simulink model "s6_template"  (R2023b)
settings: Solver=ode4  StartTime=0.0  StopTime=inf  FixedStep=P_sim_dt  RelTol=1e-3
InitFcn:
  | s6_data;
values from neighbouring files (symbols this model uses):
  CarInputsCmdForward = uint8(1)    [p_mad_car.m]
  CarInputsCmdHalt = uint8(0)    [p_mad_car.m]
  CarInputsCmdReverse = uint8(2)    [p_mad_car.m]
  CarInputsCmdSlow = uint8(3)    [p_mad_car.m]
  P_p_Bf = 0.7    [p_mad_car.m]
  P_p_Br = 0.7    [p_mad_car.m]
  P_p_Cf = 2    [p_mad_car.m]
  P_p_Cr = 2    [p_mad_car.m]
  P_p_delta_max = 21.58/180*pi    (= 0.37664205258)    [p_mad_car.m]
  P_p_Df = 2    [p_mad_car.m]
  P_p_Dr = 2.5    [p_mad_car.m]
  P_p_Ef = -0.1    [p_mad_car.m]
  P_p_Er = -0.05    [p_mad_car.m]
  P_p_J = 192e-6    (= 0.000192)    [p_mad_car.m]
  P_p_k = 2.51    [p_mad_car.m]
  P_p_l = abs(P_p_frontaxle_1 + P_p_rearaxle_1)    [p_mad_car.m]
  P_p_lf = P_p_frontaxle_1    (= 0.05)    [p_mad_car.m]
  P_p_lr = P_p_rearaxle_1    (= 0.049)    [p_mad_car.m]
  P_p_m = 132e-3    (= 0.132)    [p_mad_car.m]
  P_p_T = 316e-3    (= 0.316)    [p_mad_car.m]
  P_p_Tt = P_p_uTt + P_p_output_Tt    (= 0.1)    [p_mad_car.m]
libraries: mad_lib_template x1
settings Model: Creator=hmekiedj  LastModifiedBy=Dominik
settings SolverCC: AlgebraicLoopSolver=TrustRegion
settings DataIOCC: ReturnWorkspaceOutputs=off
settings DebuggingCC: UnconnectedInputMsg=warning  UnconnectedOutputMsg=warning  UnconnectedLineMsg=warning  ArithmeticOperatorsInVariantConditions=warning
settings ModelReferenceCC: EnableRefExpFcnMdlSchedulingChecks=on
settings SFSimCC: SimUseLocalCustomCode=off  CustomCodeUndefinedFunction=UseInterfaceOnly
settings RTWCC: RTWUseLocalCustomCode=off  DLArmComputeVersion=19.05
settings CodeAppCC: StateflowObjectComments=on

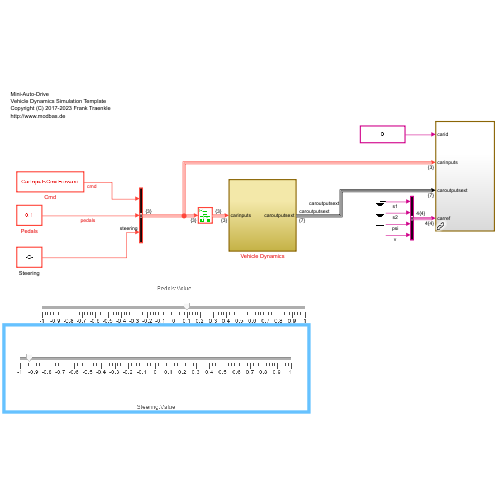
[thumbnail: Simulink's stored preview of the top-level diagram]
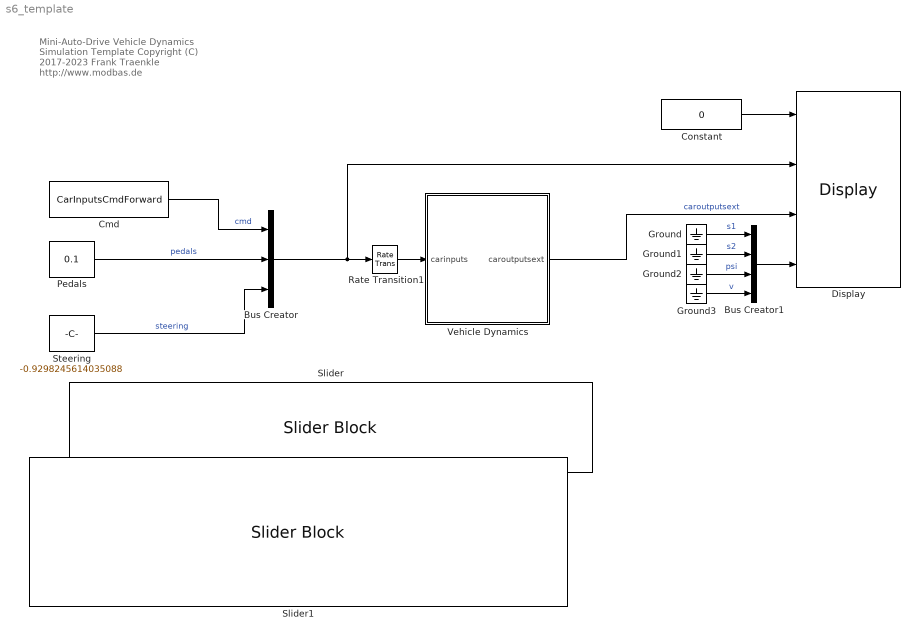
== system s6_template ==
  note: Mini-Auto-Drive
      | Vehicle Dynamics Simulation Template
      | Copyright (C) 2017-2023 Frank Traenkle
      | http://www.modbas.de
  Bus Creator : BusCreator  Inputs=3
  Bus Creator1 : BusCreator  Inputs=4
  Cmd : Constant  Value=CarInputsCmdForward  SampleTime=-1
  Constant : Constant  Value=0
  Display : mad_lib_template/Display  SystemSampleTime=-1  VariantActivationTime=update diagram  AllowFlexibleInterface=on  Latency=0  AutoFrameSizeCalculation=off
  Ground{,1..3} (4 alike) : Ground
  Pedals : Constant  Value=0.1  SampleTime=-1
  Rate Transition1 : RateTransition
  Slider : SliderBlock  ScaleMin=-1  ScaleMax=1
  Slider1 : SliderBlock  LabelPosition=Bottom  ScaleMin=-1  ScaleMax=1
  Steering : Constant  Value=-0.9298245614035088  SampleTime=-1
  Vehicle Dynamics : Subsystem
  wires:
  Pedals/1 -> Bus Creator/2  "pedals"
  Bus Creator1/1 -> Display/4
  Ground/1 -> Bus Creator1/1  "s1"
  Ground1/1 -> Bus Creator1/2  "s2"
  Ground2/1 -> Bus Creator1/3  "psi"
  Ground3/1 -> Bus Creator1/4  "v"
  Vehicle Dynamics/1(caroutputsext) -> Display/3  "caroutputsext"
  Steering/1 -> Bus Creator/3  "steering"
  Bus Creator/1 -> Display/2, Rate Transition1/1
  Rate Transition1/1 -> Vehicle Dynamics/1(carinputs)
  Constant/1 -> Display/1
  Cmd/1 -> Bus Creator/1  "cmd"

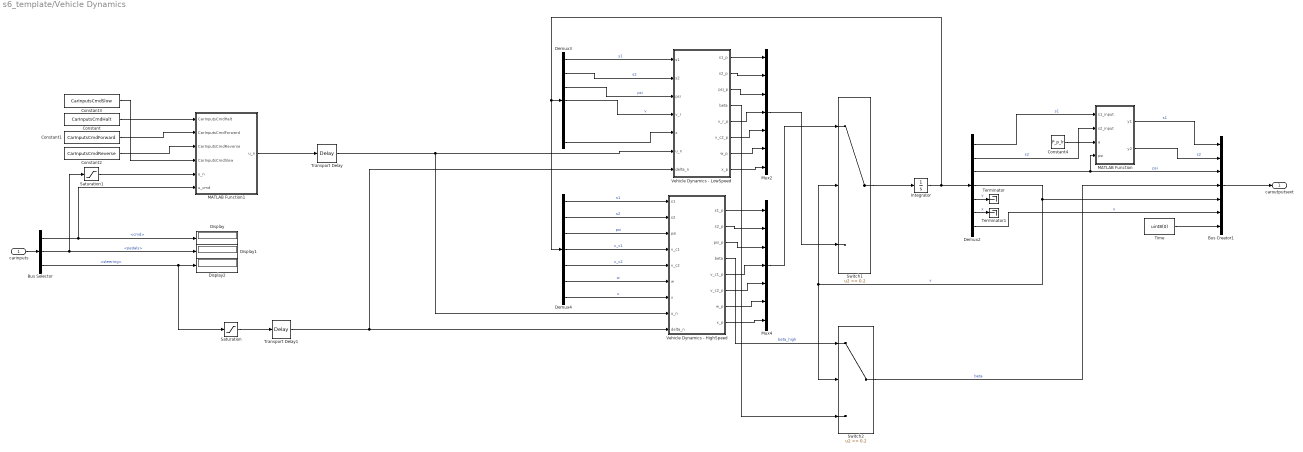
== system s6_template/Vehicle Dynamics ==
  carinputs : Inport
  Bus Creator1 : BusCreator  Inputs=7  OutDataTypeStr=Bus: CAROUTPUTSEXT
  Bus Selector : BusSelector  OutputSignals=cmd,pedals,steering
  Constant : Constant  Value=CarInputsCmdHalt
  Constant1 : Constant  Value=CarInputsCmdForward
  Constant2 : Constant  Value=CarInputsCmdReverse
  Constant3 : Constant  Value=CarInputsCmdSlow
  Constant4 : Constant  Value=P_p_lr
  Demux2 : Demux  Outputs=7
  Demux3 : Demux  Outputs=7
  Demux4 : Demux  Outputs=7
  Display : Display
  Display1 : Display
  Display2 : Display
  Integrator : Integrator
  MATLAB Function : MATLAB Function  TreatAsAtomicUnit=on
  MATLAB Function1 : MATLAB Function  TreatAsAtomicUnit=on
  Mux2 : Mux  Inputs=7
  Mux4 : Mux  Inputs=7
  Saturation : Saturate  UpperLimit=1  LowerLimit=-1
  Saturation1 : Saturate  UpperLimit=1  LowerLimit=-1
  Switch1 : Switch  Threshold=0.2  SaturateOnIntegerOverflow=off  InputSameDT=off
  Switch2 : Switch  Threshold=0.2  SaturateOnIntegerOverflow=off  InputSameDT=off
  Terminator : Terminator
  Terminator1 : Terminator
  Time : Constant  Value=uint8(0)
  Transport Delay : TransportDelay  DelayTime=P_p_Tt
  Transport Delay1 : TransportDelay  DelayTime=P_p_Tt
  Vehicle Dynamics - HighSpeed : Subsystem
  Vehicle Dynamics - LowSpeed : Subsystem
  caroutputsext : Outport  VectorParamsAs1DForOutWhenUnconnected=off
  wires:
  carinputs/1 -> Bus Selector/1
  Bus Selector/2 -> Display1/1, Saturation1/1  "<pedals>"
  Bus Selector/3 -> Saturation/1, Display2/1  "<steering>"
  Demux2/3 -> Bus Creator1/3, MATLAB Function/4(psi)  "psi"
  Bus Creator1/1 -> caroutputsext/1
  Demux2/7 -> Bus Creator1/6  "x"
  Demux2/2 -> MATLAB Function/2(s2_input)  "s2"
  Demux2/1 -> MATLAB Function/1(s1_input)  "s1"
  Bus Selector/1 -> Display/1, MATLAB Function1/6(u_cmd)  "<cmd>"
  Saturation1/1 -> MATLAB Function1/5("u_n ")
  Constant/1 -> MATLAB Function1/1(CarInputsCmdHalt)
  Constant1/1 -> MATLAB Function1/2(CarInputsCmdForward)
  Constant2/1 -> MATLAB Function1/3(CarInputsCmdReverse)
  Time/1 -> Bus Creator1/7
  Constant3/1 -> MATLAB Function1/4(CarInputsCmdSlow)
  Saturation/1 -> Transport Delay1/1
  MATLAB Function1/1(u_n) -> Transport Delay/1
  Vehicle Dynamics - HighSpeed/1(s1_p) -> Mux4/1
  Vehicle Dynamics - HighSpeed/2(s2_p) -> Mux4/2
  Vehicle Dynamics - HighSpeed/3(psi_p) -> Mux4/3
  Vehicle Dynamics - HighSpeed/5(v_c1_p) -> Mux4/4
  Vehicle Dynamics - HighSpeed/6(v_c2_p) -> Mux4/5
  Vehicle Dynamics - HighSpeed/7(w_p) -> Mux4/6
  Vehicle Dynamics - HighSpeed/8(x_p) -> Mux4/7
  Vehicle Dynamics - LowSpeed/1(s1_p) -> Mux2/1
  Vehicle Dynamics - LowSpeed/2(s2_p) -> Mux2/2
  Vehicle Dynamics - LowSpeed/3(psi_p) -> Mux2/3
  Vehicle Dynamics - LowSpeed/5(v_r_p) -> Mux2/4
  Vehicle Dynamics - LowSpeed/6(v_c2_p) -> Mux2/5
  Vehicle Dynamics - LowSpeed/7(w_p) -> Mux2/6
  Vehicle Dynamics - LowSpeed/8(x_p) -> Mux2/7
  Mux2/1 -> Switch1/3
  Mux4/1 -> Switch1/1
  Switch1/1 -> Integrator/1
  Integrator/1 -> Demux4/1, Demux3/1, Demux2/1
  Demux2/4 -> Switch2/2, Switch1/2, Bus Creator1/5  "v"
  Demux3/1 -> Vehicle Dynamics - LowSpeed/1(s1)  "s1"
  Demux3/2 -> Vehicle Dynamics - LowSpeed/2(s2)  "s2"
  Demux3/3 -> Vehicle Dynamics - LowSpeed/3(psi)  "psi"
  Demux3/4 -> Vehicle Dynamics - LowSpeed/4(v_r)  "v"
  Demux3/7 -> Vehicle Dynamics - LowSpeed/5(x)
  Demux4/1 -> Vehicle Dynamics - HighSpeed/1(s1)  "s1"
  Demux4/2 -> Vehicle Dynamics - HighSpeed/2(s2)  "s2"
  Demux4/3 -> Vehicle Dynamics - HighSpeed/3(psi)  "psi"
  Demux4/4 -> Vehicle Dynamics - HighSpeed/4(v_c1)  "v_c1"
  Demux4/5 -> Vehicle Dynamics - HighSpeed/5(v_c2)  "v_c2"
  Demux4/6 -> Vehicle Dynamics - HighSpeed/6(w)  "w"
  Demux4/7 -> Vehicle Dynamics - HighSpeed/7(x)  "x"
  Transport Delay/1 -> Vehicle Dynamics - LowSpeed/6(u_n), Vehicle Dynamics - HighSpeed/8(u_n)
  Transport Delay1/1 -> Vehicle Dynamics - LowSpeed/7(delta_n), Vehicle Dynamics - HighSpeed/9(delta_n)
  Vehicle Dynamics - LowSpeed/4(beta) -> Switch2/3
  Vehicle Dynamics - HighSpeed/4(beta) -> Switch2/1  "beta_high"
  Switch2/1 -> Bus Creator1/4  "beta"
  Constant4/1 -> MATLAB Function/3(a)
  MATLAB Function/1(y1) -> Bus Creator1/1  "s1"
  MATLAB Function/2(y2) -> Bus Creator1/2  "s2"
  Demux2/5 -> Terminator/1  "v"
  Demux2/6 -> Terminator1/1  "x"

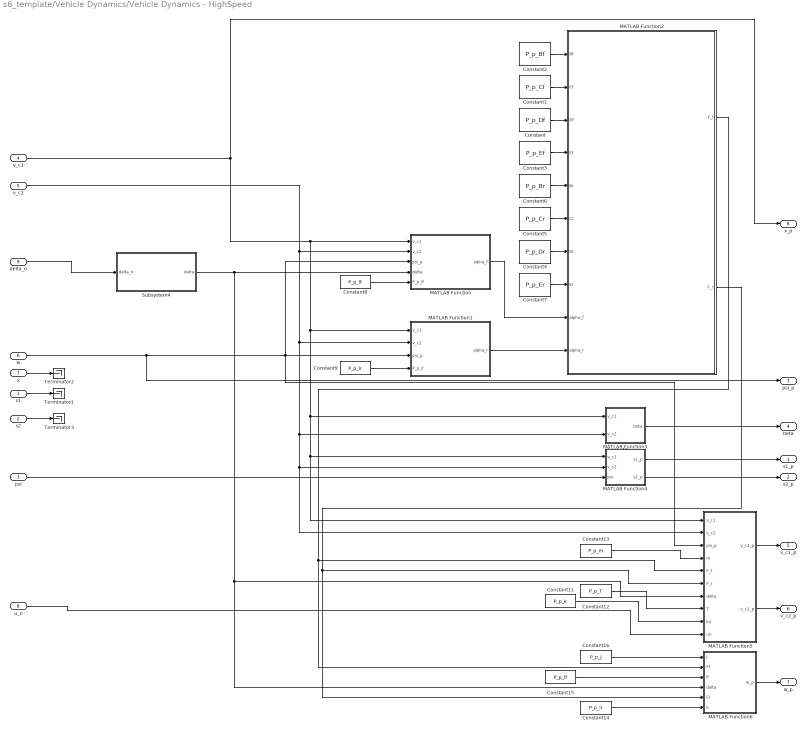
== system s6_template/Vehicle Dynamics/Vehicle Dynamics - HighSpeed ==
  s1 : Inport
  s2 : Inport  Port=2
  psi : Inport  Port=3
  v_c1 : Inport  Port=4
  v_c2 : Inport  Port=5
  w : Inport  Port=6
  x : Inport  Port=7
  u_n : Inport  Port=8
  delta_n : Inport  Port=9
  Constant : Constant  Value=P_p_Df
  Constant1 : Constant  Value=P_p_Cf
  Constant11 : Constant  Value=P_p_k
  Constant12 : Constant  Value=P_p_T
  Constant13 : Constant  Value=P_p_m
  Constant14 : Constant  Value=P_p_lr
  Constant15 : Constant  Value=P_p_lf
  Constant16 : Constant  Value=P_p_J
  Constant2 : Constant  Value=P_p_Bf
  Constant3 : Constant  Value=P_p_Ef
  Constant4 : Constant  Value=P_p_Dr
  Constant5 : Constant  Value=P_p_Cr
  Constant6 : Constant  Value=P_p_Br
  Constant7 : Constant  Value=P_p_Er
  Constant8 : Constant  Value=P_p_lf
  Constant9 : Constant  Value=P_p_lr
  MATLAB Function : MATLAB Function  TreatAsAtomicUnit=on
  MATLAB Function1 : MATLAB Function  TreatAsAtomicUnit=on
  MATLAB Function2 : MATLAB Function  TreatAsAtomicUnit=on
  MATLAB Function3 : MATLAB Function  TreatAsAtomicUnit=on
  MATLAB Function4 : MATLAB Function  TreatAsAtomicUnit=on
  MATLAB Function5 : MATLAB Function  TreatAsAtomicUnit=on
  MATLAB Function6 : MATLAB Function  TreatAsAtomicUnit=on
  Subsystem4 : Subsystem
  Terminator1 : Terminator
  Terminator2 : Terminator
  Terminator3 : Terminator
  s1_p : Outport  VectorParamsAs1DForOutWhenUnconnected=off
  s2_p : Outport  Port=2  VectorParamsAs1DForOutWhenUnconnected=off
  psi_p : Outport  Port=3  VectorParamsAs1DForOutWhenUnconnected=off
  beta : Outport  Port=4  VectorParamsAs1DForOutWhenUnconnected=off
  v_c1_p : Outport  Port=5  VectorParamsAs1DForOutWhenUnconnected=off
  v_c2_p : Outport  Port=6  VectorParamsAs1DForOutWhenUnconnected=off
  w_p : Outport  Port=7  VectorParamsAs1DForOutWhenUnconnected=off
  x_p : Outport  Port=8  VectorParamsAs1DForOutWhenUnconnected=off
  wires:
  delta_n/1 -> Subsystem4/1(delta_n)
  Constant2/1 -> MATLAB Function2/1(Bf)
  Constant1/1 -> MATLAB Function2/2(Cf)
  Constant/1 -> MATLAB Function2/3(Df)
  Constant3/1 -> MATLAB Function2/4(Ef)
  Constant6/1 -> MATLAB Function2/5(Br)
  Constant5/1 -> MATLAB Function2/6(Cr)
  Constant4/1 -> MATLAB Function2/7(Dr)
  Constant7/1 -> MATLAB Function2/8(Er)
  MATLAB Function/1(alpha_f) -> MATLAB Function2/9(alpha_f)
  MATLAB Function1/1(alpha_r) -> MATLAB Function2/10(alpha_r)
  MATLAB Function3/1(beta) -> beta/1
  MATLAB Function4/1(s1_p) -> s1_p/1
  MATLAB Function4/2(s2_p) -> s2_p/1
  Subsystem4/1(delta) -> MATLAB Function/4(delta), MATLAB Function5/7(delta), MATLAB Function6/4(delta)
  Constant8/1 -> MATLAB Function/5(P_p_lf)
  Constant9/1 -> MATLAB Function1/4(P_p_lr)
  w/1 -> MATLAB Function1/3(psi_p), MATLAB Function/3(psi_p), MATLAB Function5/3(psi_p), psi_p/1
  u_n/1 -> MATLAB Function5/10(un)
  Constant11/1 -> MATLAB Function5/9(ku)
  Constant12/1 -> MATLAB Function5/8(T)
  MATLAB Function2/2(F_r) -> MATLAB Function5/6(F_r), MATLAB Function6/5(Fr)
  MATLAB Function2/1(F_f) -> MATLAB Function5/5(F_f), MATLAB Function6/2(Ff)
  MATLAB Function5/1(v_c1_p) -> v_c1_p/1
  MATLAB Function5/2(v_c2_p) -> v_c2_p/1
  Constant13/1 -> MATLAB Function5/4(m)
  v_c1/1 -> MATLAB Function/1(v_c1), MATLAB Function5/1(v_c1), MATLAB Function4/1(v_c1), MATLAB Function3/1(v_c1), MATLAB Function1/1(v_c1), x_p/1
  v_c2/1 -> MATLAB Function/2(v_c2), MATLAB Function5/2(v_c2), MATLAB Function4/2(v_c2), MATLAB Function3/2(v_c2), MATLAB Function1/2(v_c2)
  Constant14/1 -> MATLAB Function6/6(lr)
  Constant15/1 -> MATLAB Function6/3(lf)
  Constant16/1 -> MATLAB Function6/1(J)
  MATLAB Function6/1(w_p) -> w_p/1
  psi/1 -> MATLAB Function4/3(psi)
  x/1 -> Terminator2/1
  s1/1 -> Terminator1/1
  s2/1 -> Terminator3/1

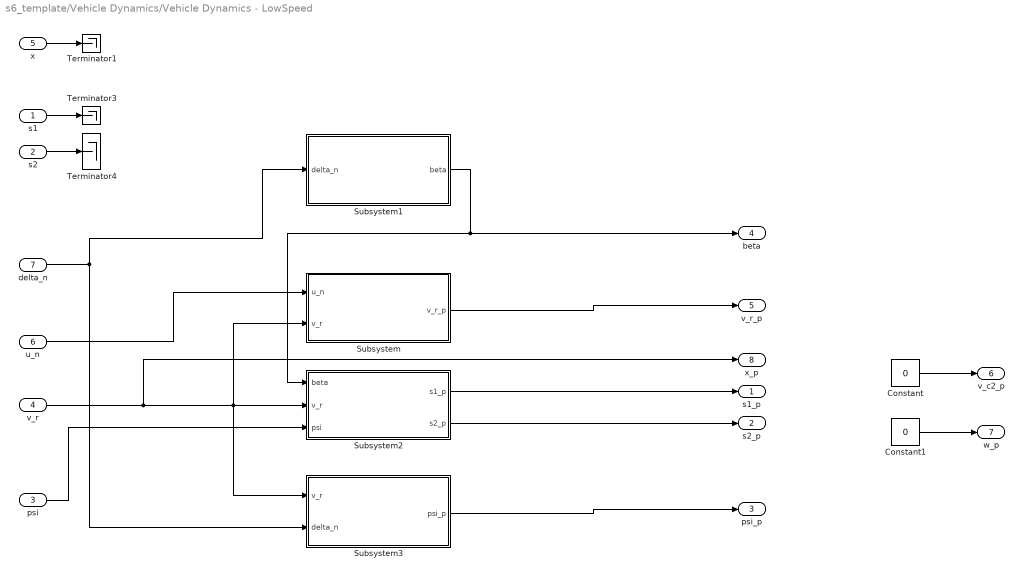
== system s6_template/Vehicle Dynamics/Vehicle Dynamics - LowSpeed ==
  s1 : Inport
  s2 : Inport  Port=2
  psi : Inport  Port=3
  v_r : Inport  Port=4
  x : Inport  Port=5
  u_n : Inport  Port=6
  delta_n : Inport  Port=7
  Constant : Constant  Value=0
  Constant1 : Constant  Value=0
  Subsystem : Subsystem
  Subsystem1 : Subsystem
  Subsystem2 : Subsystem
  Subsystem3 : Subsystem
  Terminator1 : Terminator
  Terminator3 : Terminator
  Terminator4 : Terminator
  s1_p : Outport  VectorParamsAs1DForOutWhenUnconnected=off
  s2_p : Outport  Port=2  VectorParamsAs1DForOutWhenUnconnected=off
  psi_p : Outport  Port=3  VectorParamsAs1DForOutWhenUnconnected=off
  beta : Outport  Port=4  VectorParamsAs1DForOutWhenUnconnected=off
  v_r_p : Outport  Port=5  VectorParamsAs1DForOutWhenUnconnected=off
  v_c2_p : Outport  Port=6  VectorParamsAs1DForOutWhenUnconnected=off
  w_p : Outport  Port=7  VectorParamsAs1DForOutWhenUnconnected=off
  x_p : Outport  Port=8  VectorParamsAs1DForOutWhenUnconnected=off
  wires:
  u_n/1 -> Subsystem/1(u_n)
  Subsystem/1(v_r_p) -> v_r_p/1
  v_r/1 -> x_p/1, Subsystem3/1(v_r), Subsystem2/2(v_r), Subsystem/2(v_r)
  delta_n/1 -> Subsystem3/2(delta_n), Subsystem1/1(delta_n)
  Subsystem2/1(s1_p) -> s1_p/1
  psi/1 -> Subsystem2/3(psi)
  Subsystem1/1(beta) -> Subsystem2/1(beta), beta/1
  Subsystem2/2(s2_p) -> s2_p/1
  Subsystem3/1(psi_p) -> psi_p/1
  x/1 -> Terminator1/1
  s1/1 -> Terminator3/1
  s2/1 -> Terminator4/1
  Constant/1 -> v_c2_p/1
  Constant1/1 -> w_p/1

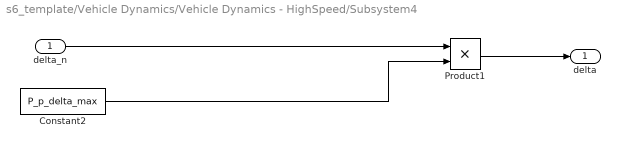
== system s6_template/Vehicle Dynamics/Vehicle Dynamics - HighSpeed/Subsystem4 ==
  delta_n : Inport
  Constant2 : Constant  Value=P_p_delta_max
  Product1 : Product
  delta : Outport  VectorParamsAs1DForOutWhenUnconnected=off
  wires:
  delta_n/1 -> Product1/1
  Constant2/1 -> Product1/2
  Product1/1 -> delta/1

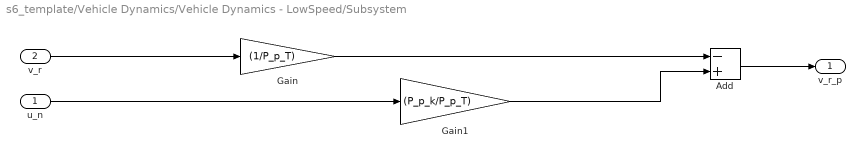
== system s6_template/Vehicle Dynamics/Vehicle Dynamics - LowSpeed/Subsystem ==
  u_n : Inport
  v_r : Inport  Port=2
  Add : Sum  Inputs=-+
  Gain : Gain  Gain=(1/P_p_T)
  Gain1 : Gain  Gain=(P_p_k/P_p_T)
  v_r_p : Outport  VectorParamsAs1DForOutWhenUnconnected=off
  wires:
  Gain/1 -> Add/1
  Add/1 -> v_r_p/1
  v_r/1 -> Gain/1
  u_n/1 -> Gain1/1
  Gain1/1 -> Add/2

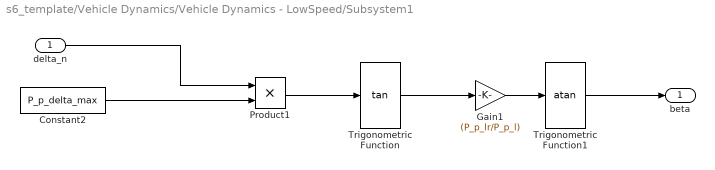
== system s6_template/Vehicle Dynamics/Vehicle Dynamics - LowSpeed/Subsystem1 ==
  delta_n : Inport
  Constant2 : Constant  Value=P_p_delta_max
  Gain1 : Gain  Gain=(P_p_lr/P_p_l)
  Product1 : Product
  Trigonometric Function : Trigonometry  Operator=tan
  Trigonometric Function1 : Trigonometry  Operator=atan
  beta : Outport  VectorParamsAs1DForOutWhenUnconnected=off
  wires:
  delta_n/1 -> Product1/1
  Constant2/1 -> Product1/2
  Product1/1 -> Trigonometric Function/1
  Trigonometric Function/1 -> Gain1/1
  Gain1/1 -> Trigonometric Function1/1
  Trigonometric Function1/1 -> beta/1

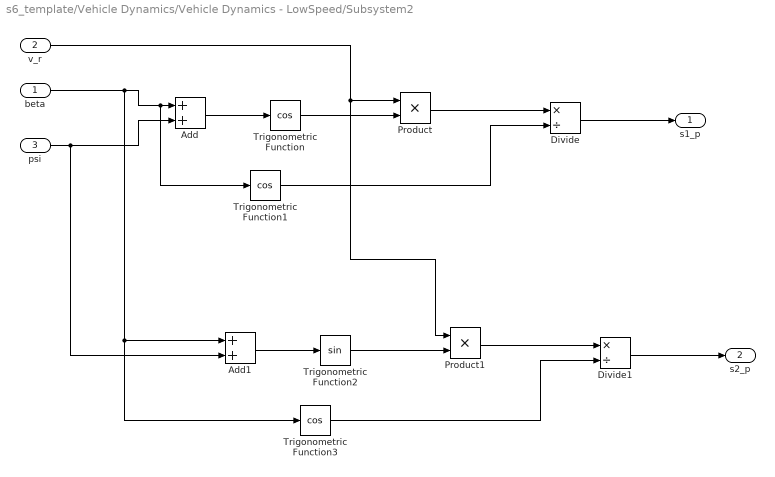
== system s6_template/Vehicle Dynamics/Vehicle Dynamics - LowSpeed/Subsystem2 ==
  beta : Inport
  v_r : Inport  Port=2
  psi : Inport  Port=3
  Add : Sum
  Add1 : Sum
  Divide : Product  Inputs=*/
  Divide1 : Product  Inputs=*/
  Product : Product
  Product1 : Product
  Trigonometric Function : Trigonometry  Operator=cos
  Trigonometric Function1 : Trigonometry  Operator=cos
  Trigonometric Function2 : Trigonometry
  Trigonometric Function3 : Trigonometry  Operator=cos
  s1_p : Outport  VectorParamsAs1DForOutWhenUnconnected=off
  s2_p : Outport  Port=2  VectorParamsAs1DForOutWhenUnconnected=off
  wires:
  Add/1 -> Trigonometric Function/1
  Trigonometric Function/1 -> Product/2
  Product/1 -> Divide/1
  Trigonometric Function1/1 -> Divide/2
  Divide/1 -> s1_p/1
  psi/1 -> Add/2, Add1/2
  beta/1 -> Add1/1, Trigonometric Function3/1, Trigonometric Function1/1, Add/1
  Trigonometric Function2/1 -> Product1/2
  Divide1/1 -> s2_p/1
  v_r/1 -> Product1/1, Product/1
  Product1/1 -> Divide1/1
  Add1/1 -> Trigonometric Function2/1
  Trigonometric Function3/1 -> Divide1/2

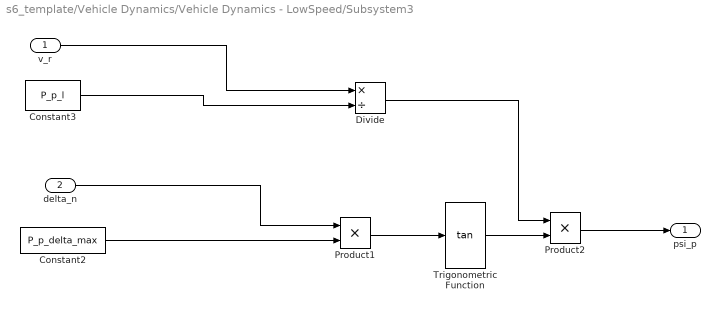
== system s6_template/Vehicle Dynamics/Vehicle Dynamics - LowSpeed/Subsystem3 ==
  v_r : Inport
  delta_n : Inport  Port=2
  Constant2 : Constant  Value=P_p_delta_max
  Constant3 : Constant  Value=P_p_l
  Divide : Product  Inputs=*/
  Product1 : Product
  Product2 : Product
  Trigonometric Function : Trigonometry  Operator=tan
  psi_p : Outport  VectorParamsAs1DForOutWhenUnconnected=off
  wires:
  delta_n/1 -> Product1/1
  Constant2/1 -> Product1/2
  Product1/1 -> Trigonometric Function/1
  Product2/1 -> psi_p/1
  v_r/1 -> Divide/1
  Constant3/1 -> Divide/2
  Trigonometric Function/1 -> Product2/2
  Divide/1 -> Product2/1

== matlab function s6_template/Vehicle Dynamics/Vehicle Dynamics - HighSpeed/MATLAB Function5 ==
  data: v_c1 input; v_c1_p output; v_c2 input; psi_p input; v_c2_p output; m input; F_f input; F_r input; delta input; T input; ku input; un input
function [v_c1_p, v_c2_p] = fcn(v_c1,v_c2,psi_p,m,F_f,F_r,delta,T,ku,un)
v_c1_p = double((1/m) * (-F_f * sin(delta) + (m*v_c2*psi_p)) - (1/T*v_c1) + ((ku/T)*un));
v_c2_p = double((1/m) * (F_f * cos(delta) + F_r - (m * v_c1 * psi_p)));

== matlab function s6_template/Vehicle Dynamics/Vehicle Dynamics - HighSpeed/MATLAB Function6 ==
  data: J input; w_p output; Ff input; lf input; delta input; Fr input; lr input
function w_p = fcn(J,Ff,lf,delta,Fr,lr)
w_p = 1/J * (Ff*lf*cos(delta)-Fr*lr);

== matlab function s6_template/Vehicle Dynamics/MATLAB Function1 ==
  data: CarInputsCmdHalt input; CarInputsCmdForward input; CarInputsCmdReverse input; CarInputsCmdSlow input; u_n input; u_n output; u_cmd input
function u_n = fcn(CarInputsCmdHalt, CarInputsCmdForward, CarInputsCmdReverse,CarInputsCmdSlow, u_n, u_cmd)

if (u_cmd == CarInputsCmdHalt)
    u_n = 0;
elseif (u_cmd == CarInputsCmdForward && u_n < 0)
    u_n = 0;
elseif (u_cmd == CarInputsCmdReverse && u_n > 0)
    u_n = 0;
elseif u_cmd == CarInputsCmdForward && u_n > 1
    u_n = 1;
elseif u_cmd == CarInputsCmdReverse && u_n < -1
    u_n = -1;
else
    u_n = u_n;
end

== matlab function s6_template/Vehicle Dynamics/MATLAB Function ==
  data: s1_input input; y1 output; s2_input input; a input; psi input; y2 output
function [y1,y2] = fcn(s1_input,s2_input,a,psi)

y1=s1_input-(a*cos(psi));
y2=s2_input-(a*sin(psi));

== matlab function s6_template/Vehicle Dynamics/Vehicle Dynamics - HighSpeed/MATLAB Function1 ==
  data: v_c1 input; alpha_r output; v_c2 input; psi_p input; P_p_lr input
function alpha_r = fcn(v_c1,v_c2,psi_p,P_p_lr)
if (v_c1>0)
    alpha_r = -atan((v_c2-(P_p_lr*psi_p))/(v_c1));
elseif (v_c1<0)
    alpha_r = atan((v_c2-(P_p_lr*psi_p))/(v_c1));
else 
    alpha_r = 0;
end

== matlab function s6_template/Vehicle Dynamics/Vehicle Dynamics - HighSpeed/MATLAB Function ==
  data: v_c1 input; alpha_f output; v_c2 input; psi_p input; delta input; P_p_lf input
function alpha_f = fcn(v_c1,v_c2,psi_p,delta,P_p_lf)
if (v_c1 > 0)
    alpha_f = -atan((v_c2+(P_p_lf*psi_p))/(v_c1))+delta;
elseif (v_c1 < 0)
    alpha_f = atan((v_c2+(P_p_lf*psi_p))/(v_c1))-delta;
else
    alpha_f = 0;
end

== matlab function s6_template/Vehicle Dynamics/Vehicle Dynamics - HighSpeed/MATLAB Function2 ==
  data: Bf input; F_f output; Cf input; Df input; Ef input; Br input; Cr input; Dr input; Er input; alpha_f input; alpha_r input; F_r output
function [F_f,F_r] = fcn(Bf,Cf,Df,Ef,Br,Cr,Dr,Er,alpha_f,alpha_r)
    F_f = Df * sin(Cf*atan(Bf*(1-Ef)*alpha_f-(Ef*atan(Bf*alpha_f))));
    F_r = Dr * sin(Cr*atan(Br*(1-Er)*alpha_r-(Er*atan(Br*alpha_r))));
end

== matlab function s6_template/Vehicle Dynamics/Vehicle Dynamics - HighSpeed/MATLAB Function3 ==
  data: v_c1 input; beta output; v_c2 input
function beta = fcn(v_c1,v_c2)
beta = atan2(v_c2,v_c1);

== matlab function s6_template/Vehicle Dynamics/Vehicle Dynamics - HighSpeed/MATLAB Function4 ==
  data: v_c1 input; s1_p output; v_c2 input; psi input; s2_p output
function [s1_p,s2_p] = fcn(v_c1,v_c2,psi)
s1_p = v_c1*cos(psi) - v_c2*sin(psi);
s2_p = v_c1*sin(psi) + v_c2*cos(psi);
